simulink model "HDVSim_BEV_Truck"  (R2019b)
settings: Solver=ode3  StartTime=0.0  StopTime=inf  FixedStep=sample_time  MaxStep=0.1  RelTol=1e-3  EnableMultiTasking=on
model workspace (MAT data in the model file):
  Bat : object (value not decoded)
  Electric_Truck = 1
  FuelCell : P_nom (value not decoded)
  Fueltype = 7
  Hybrid_Truck = 1
  IZ12 = 3600
  M_el = 1000
  SOC_T_EM_completely_available = 0.5
  SOC_addition = 0.4
  SOC_el = 0.8
  SOC_target = 0.85
  Sailing_without_drag_torque = 0
  TCO : object (value not decoded)
  TCO_Trailer = 1
  T_distance_LPS_down = 250
  T_distance_LPS_up = 250
  VSim : object (value not decoded)
  Vehicle = 'empty'
  WPT : object (value not decoded)
  acquisitionCosts : acquisitionCosts (value not decoded)
  addition_for_critical_slope = 0.01
  ambient : object (value not decoded)
  auxiliary_consumers : object (value not decoded)
  critical_altitude_difference = 50
  cycle : object (value not decoded)
  dcycle = 22
  distance_1_PPC = 175
  distance_2_PPC = 200
  distance_PPC_altitude_difference = 10000
  driver : object (value not decoded)
  em : object (value not decoded)
  engine : object (value not decoded)
  final_drive : object (value not decoded)
  ifElectric = 1
  ifOptimized = 0
  look_ahead_PPC = 250
  max_distance = 100000
  name = 'HDVSim_BEV_Truck'
  preditiveCruiseControl = 0
  sample_time = 0.1
  tank : object (value not decoded)
  tires : object (value not decoded)
  transmission : object (value not decoded)
  v_PPC_delta = 2.77777777778
  v_max_electrical_drive_only = 13.8888888889
  vehicle : object (value not decoded)
  vehicleProperties : vehicleProperties (value not decoded)
  weights : weights (value not decoded)
  x = 1
values from neighbouring files (symbols this model uses):
  transmission = Transmission_gearing(15.86, 7, 0, 0, final_drive.ratio)    [Parameterizing.m]
symbols that are objects in the model workspace (value not decoded): ambient, auxiliary_consumers, Bat, cycle, driver, em, final_drive, tires, vehicle
undefined symbols (not defined in the file or in its folder): Ion, Lithium, prospective_cruise_control, Vorausschauender_Tempomat
libraries: simulink x21, powerlib x2, electricdrivelib x1
(part 2 of 3)

== system HDVSim_BEV_Truck/Active cruise control1/Estimate acceleration ==
  v_target [m/s] : Inport
  Slope_0 : Inport  Port=2
  Slope_50 : Inport  Port=3
  Slope_100 : Inport  Port=4
  Slope_150 : Inport  Port=5
  Slope_200 : Inport  Port=6
  "Slope_250 " : Inport  Port=7
  Slope_300 : Inport  Port=8
  Slope_350 : Inport  Port=9
  Slope_400 : Inport  Port=10
  Slope_450 : Inport  Port=11
  Add4 : Sum
  Constant4 : Constant  Value=vehicle.payload
  Constant9 : Constant  Value=vehicle.mass
  Demux : Demux  Outputs=10
  Divide1 : Product  Inputs=*/
  Driving resistance without acceleration : Subsystem
  Gain1 : Gain  Gain=-1
  Mux : Mux  Inputs=10
  Trigonometric Function2 : Trigonometry  Operator=atan
  Acceleration_0 : Outport  VectorParamsAs1DForOutWhenUnconnected=off
  Acceleration_50 : Outport  Port=2  VectorParamsAs1DForOutWhenUnconnected=off
  Acceleration_100 : Outport  Port=3  VectorParamsAs1DForOutWhenUnconnected=off
  Acceleration_150 : Outport  Port=4  VectorParamsAs1DForOutWhenUnconnected=off
  Acceleration_200 : Outport  Port=5  VectorParamsAs1DForOutWhenUnconnected=off
  Acceleration_250 : Outport  Port=6  VectorParamsAs1DForOutWhenUnconnected=off
  Acceleration_300 : Outport  Port=7  VectorParamsAs1DForOutWhenUnconnected=off
  Acceleration_350 : Outport  Port=8  VectorParamsAs1DForOutWhenUnconnected=off
  Acceleration_400 : Outport  Port=9  VectorParamsAs1DForOutWhenUnconnected=off
  Acceleration_450 : Outport  Port=10  VectorParamsAs1DForOutWhenUnconnected=off
  wires:
  v_target [m/s]/1 -> Driving resistance without acceleration/1(v [m/s])
  Trigonometric Function2/1 -> Driving resistance without acceleration/2(alpha [rad])
  Constant9/1 -> Add4/1
  Constant4/1 -> Add4/2
  Driving resistance without acceleration/1(F_x (resist) [N]) -> Gain1/1
  Add4/1 -> Divide1/2
  Gain1/1 -> Divide1/1
  Mux/1 -> Trigonometric Function2/1
  Divide1/1 -> Demux/1
  Demux/1 -> Acceleration_0/1
  Slope_0/1 -> Mux/1
  Slope_50/1 -> Mux/2
  Slope_100/1 -> Mux/3
  Slope_150/1 -> Mux/4
  Slope_200/1 -> Mux/5
  "Slope_250 "/1 -> Mux/6
  Slope_300/1 -> Mux/7
  Slope_350/1 -> Mux/8
  Slope_400/1 -> Mux/9
  Slope_450/1 -> Mux/10
  Demux/2 -> Acceleration_50/1
  Demux/3 -> Acceleration_100/1
  Demux/4 -> Acceleration_150/1
  Demux/5 -> Acceleration_200/1
  Demux/6 -> Acceleration_250/1
  Demux/7 -> Acceleration_300/1
  Demux/8 -> Acceleration_350/1
  Demux/9 -> Acceleration_400/1
  Demux/10 -> Acceleration_450/1

== system HDVSim_BEV_Truck/Active cruise control1/Estimate critical slope ==
  note: Total resistive forces on the vehicle
  note: Friction resistance
  note: Drag on the vehicle
  note: Forward force applied on the vehicle
  v_target [m/s] : Inport
  A : Constant  Value=vehicle.frontal_area
  Add : Sum
  Add1 : Sum
  Constant1 : Constant  Value=vehicle.payload
  Constant4 : Constant  Value=addition_for_critical_slope
  Constant5 : Constant  Value=tires.roll_drag_coeff.total
  Constant8 : Constant  Value=vehicle.mass
  Differential gear ratio : Constant  Value=final_drive.ratio
  Divide : Product  Inputs=***/
  Divide1 : Product  Inputs=*/
  Gain : Gain  Gain=0.95
  Product : Product
  Product2 : Product  Inputs=4  RndMeth=Zero
  Saturation : Saturate  UpperLimit=1  LowerLimit=-1
  Subtract : Sum  Inputs=+-
  Sum3 : Sum  Inputs=++|
  Tire radius : Constant  Value=tires.radius
  Trigonometric Function : Trigonometry  Operator=asin
  Trigonometric Function1 : Trigonometry  Operator=tan
  c_d : Constant  Value=vehicle.air_drag_coeff(end)
  g : Gain  Gain=ambient.gravity
  gain2 : Gain  Gain=0.5
  rho : Constant  Value=ambient.air_density
  v² : Math  Operator=square  SaturateOnIntegerOverflow=on
  critical_slope : Outport  VectorParamsAs1DForOutWhenUnconnected=off
  wires:
  Subtract/1 -> Divide1/1  "F_net"
  v²/1 -> Product2/1
  rho/1 -> Product2/2
  A/1 -> Product2/3
  c_d/1 -> Product2/4
  Product2/1 -> gain2/1
  Constant8/1 -> Add1/1
  Constant1/1 -> Add1/2
  Add1/1 -> g/1
  Constant5/1 -> Product/2
  Trigonometric Function/1 -> Trigonometric Function1/1
  Divide1/1 -> Saturation/1
  Sum3/1 -> critical_slope/1
  Constant4/1 -> Sum3/1
  Trigonometric Function1/1 -> Sum3/2
  v_target [m/s]/1 -> v²/1
  gain2/1 -> Add/1
  Product/1 -> Add/2
  Add/1 -> Subtract/2  "F_resistive"
  g/1 -> Product/1, Divide1/2
  Saturation/1 -> Trigonometric Function/1
  Tire radius/1 -> Divide/4
  Differential gear ratio/1 -> Divide/2
  Gain/1 -> Divide/3
  [i_gearbox] -> Divide/1
  Divide/1 -> Subtract/1
  [M_EM_max] -> Gain/1

== system HDVSim_BEV_Truck/Active cruise control2/Braking from upper speed limit ==
  v_target [m/s] : Inport
  Add3 : Sum  Inputs=+-
  Constant1 : Constant  Value=90/3.6
  Constant10 : Constant  Value=preditiveCruiseControl
  Constant6 : Constant  Value=v_PPC_delta
  Constant7 : Constant  Value=0
  Constant8 : Constant  Value=0
  Saturation Dynamic : simulink/Discontinuities/Saturation Dynamic  OutMin=[]  OutMax=[]  OutDataTypeStr=Inherit: Same as second input  OutDataType=fixdt(1, 16)  OutScaling=2^-10  DoSatur=off
  Switch3 : Switch  Criteria=u2 > Threshold
  Out1 : Outport  VectorParamsAs1DForOutWhenUnconnected=off
  wires:
  Switch3/1 -> Out1/1
  Constant6/1 -> Saturation Dynamic/2
  Constant1/1 -> Add3/1
  Constant7/1 -> Switch3/3
  Add3/1 -> Saturation Dynamic/1
  Constant8/1 -> Saturation Dynamic/3
  Constant10/1 -> Switch3/2
  v_target [m/s]/1 -> Add3/2
  Saturation Dynamic/1 -> Switch3/1

== system HDVSim_BEV_Truck/Active cruise control2/Estimate acceleration ==
  v_target [m/s] : Inport
  Slope_0 : Inport  Port=2
  Slope_50 : Inport  Port=3
  Slope_100 : Inport  Port=4
  Slope_150 : Inport  Port=5
  Slope_200 : Inport  Port=6
  "Slope_250 " : Inport  Port=7
  Slope_300 : Inport  Port=8
  Slope_350 : Inport  Port=9
  Slope_400 : Inport  Port=10
  Slope_450 : Inport  Port=11
  Add4 : Sum
  Constant4 : Constant  Value=vehicle.payload
  Constant9 : Constant  Value=vehicle.mass
  Demux : Demux  Outputs=10
  Divide1 : Product  Inputs=*/
  Driving resistance without acceleration : Subsystem
  Gain1 : Gain  Gain=-1
  Mux : Mux  Inputs=10
  Trigonometric Function2 : Trigonometry  Operator=atan
  Acceleration_0 : Outport  VectorParamsAs1DForOutWhenUnconnected=off
  Acceleration_50 : Outport  Port=2  VectorParamsAs1DForOutWhenUnconnected=off
  Acceleration_100 : Outport  Port=3  VectorParamsAs1DForOutWhenUnconnected=off
  Acceleration_150 : Outport  Port=4  VectorParamsAs1DForOutWhenUnconnected=off
  Acceleration_200 : Outport  Port=5  VectorParamsAs1DForOutWhenUnconnected=off
  Acceleration_250 : Outport  Port=6  VectorParamsAs1DForOutWhenUnconnected=off
  Acceleration_300 : Outport  Port=7  VectorParamsAs1DForOutWhenUnconnected=off
  Acceleration_350 : Outport  Port=8  VectorParamsAs1DForOutWhenUnconnected=off
  Acceleration_400 : Outport  Port=9  VectorParamsAs1DForOutWhenUnconnected=off
  Acceleration_450 : Outport  Port=10  VectorParamsAs1DForOutWhenUnconnected=off
  wires:
  v_target [m/s]/1 -> Driving resistance without acceleration/1(v [m/s])
  Trigonometric Function2/1 -> Driving resistance without acceleration/2(alpha [rad])
  Constant9/1 -> Add4/1
  Constant4/1 -> Add4/2
  Driving resistance without acceleration/1(F_x (resist) [N]) -> Gain1/1
  Add4/1 -> Divide1/2
  Gain1/1 -> Divide1/1
  Mux/1 -> Trigonometric Function2/1
  Divide1/1 -> Demux/1
  Demux/1 -> Acceleration_0/1
  Slope_0/1 -> Mux/1
  Slope_50/1 -> Mux/2
  Slope_100/1 -> Mux/3
  Slope_150/1 -> Mux/4
  Slope_200/1 -> Mux/5
  "Slope_250 "/1 -> Mux/6
  Slope_300/1 -> Mux/7
  Slope_350/1 -> Mux/8
  Slope_400/1 -> Mux/9
  Slope_450/1 -> Mux/10
  Demux/2 -> Acceleration_50/1
  Demux/3 -> Acceleration_100/1
  Demux/4 -> Acceleration_150/1
  Demux/5 -> Acceleration_200/1
  Demux/6 -> Acceleration_250/1
  Demux/7 -> Acceleration_300/1
  Demux/8 -> Acceleration_350/1
  Demux/9 -> Acceleration_400/1
  Demux/10 -> Acceleration_450/1

== system HDVSim_BEV_Truck/Active cruise control2/Estimate critical slope ==
  note: Total resistive forces on the vehicle
  note: Friction resistance
  note: Drag on the vehicle
  note: Forward force applied on the vehicle
  v_target [m/s] : Inport
  A : Constant  Value=vehicle.frontal_area
  Add : Sum
  Add1 : Sum
  Add3 : Sum
  Constant1 : Constant  Value=vehicle.payload
  Constant4 : Constant  Value=addition_for_critical_slope
  Constant5 : Constant  Value=tires.roll_drag_coeff.total
  Constant8 : Constant  Value=vehicle.mass
  Differential efficiency : Constant  Value=final_drive.trq_eff
  Differential gear ratio : Constant  Value=final_drive.ratio
  Divide : Product  Inputs=***/**
  Divide1 : Product  Inputs=*/
  Product : Product
  Product2 : Product  Inputs=4  RndMeth=Zero
  Subtract : Sum  Inputs=+-
  Sum3 : Sum  Inputs=++|
  Tire radius : Constant  Value=tires.radius
  Trigonometric Function : Trigonometry  Operator=asin
  Trigonometric Function1 : Trigonometry  Operator=tan
  c_d : Constant  Value=vehicle.air_drag_coeff(end)
  g : Gain  Gain=ambient.gravity
  gain2 : Gain  Gain=0.5
  rho : Constant  Value=ambient.air_density
  v² : Math  Operator=square  SaturateOnIntegerOverflow=on
  critical_slope : Outport  VectorParamsAs1DForOutWhenUnconnected=off
  wires:
  Add3/1 -> Divide/3
  [i_gearbox] -> Divide/1
  Differential gear ratio/1 -> Divide/2
  Tire radius/1 -> Divide/4
  Divide/1 -> Subtract/1
  Subtract/1 -> Divide1/1  "F_net"
  v²/1 -> Product2/1
  rho/1 -> Product2/2
  A/1 -> Product2/3
  c_d/1 -> Product2/4
  Product2/1 -> gain2/1
  Constant8/1 -> Add1/1
  Constant1/1 -> Add1/2
  Add1/1 -> g/1
  Constant5/1 -> Product/2
  Trigonometric Function/1 -> Trigonometric Function1/1
  Divide1/1 -> Trigonometric Function/1
  Sum3/1 -> critical_slope/1
  Constant4/1 -> Sum3/1
  Trigonometric Function1/1 -> Sum3/2
  v_target [m/s]/1 -> v²/1
  [Eta_Transmission] -> Divide/5
  Differential efficiency/1 -> Divide/6
  [M_EM_max] -> Add3/1
  [M_EM_max] -> Add3/2
  gain2/1 -> Add/1
  Product/1 -> Add/2
  Add/1 -> Subtract/2  "F_resistive"
  g/1 -> Product/1, Divide1/2

== system HDVSim_BEV_Truck/Active cruise control_old/Braking from upper speed limit ==
  v_soll [m/s] : Inport
  Add3 : Sum  Inputs=+-
  Constant1 : Constant  Value=90/3.6
  Constant10 : Constant  Value=Vorausschauender_Tempomat
  Constant6 : Constant  Value=6/3.6
  Constant7 : Constant  Value=0
  Constant8 : Constant  Value=0
  Saturation Dynamic : simulink/Discontinuities/Saturation Dynamic  OutMin=[]  OutMax=[]  OutDataTypeStr=Inherit: Same as second input  OutDataType=fixdt(1, 16)  OutScaling=2^-10  DoSatur=off
  Switch3 : Switch  Criteria=u2 > Threshold
  Out1 : Outport  VectorParamsAs1DForOutWhenUnconnected=off
  wires:
  Switch3/1 -> Out1/1
  Constant6/1 -> Saturation Dynamic/2
  Constant1/1 -> Add3/1
  Constant7/1 -> Switch3/3
  Add3/1 -> Saturation Dynamic/1
  Constant8/1 -> Saturation Dynamic/3
  Constant10/1 -> Switch3/2
  v_soll [m/s]/1 -> Add3/2
  Saturation Dynamic/1 -> Switch3/1

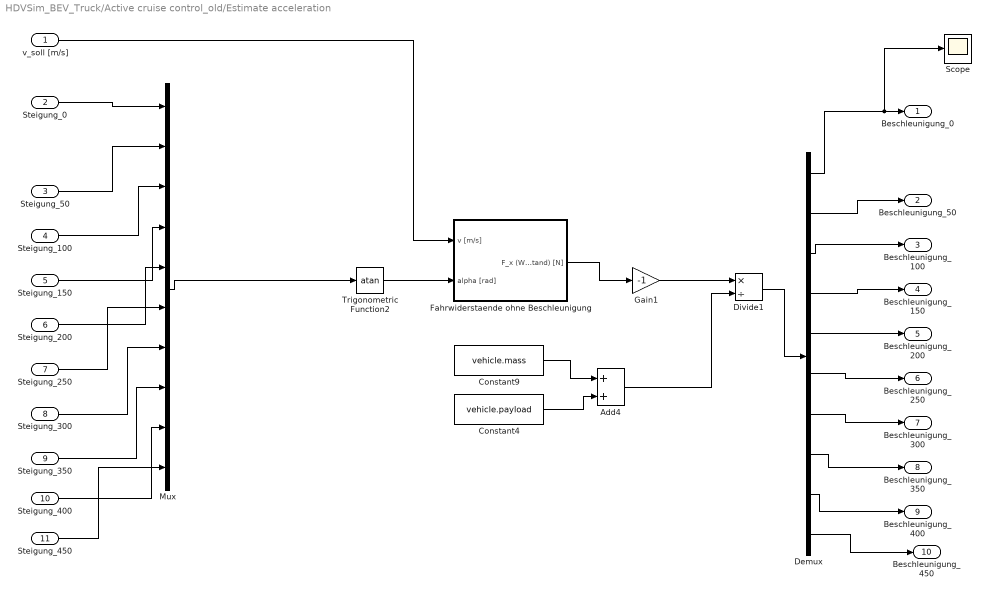
== system HDVSim_BEV_Truck/Active cruise control_old/Estimate acceleration ==
  v_soll [m/s] : Inport
  Steigung_0 : Inport  Port=2
  Steigung_50 : Inport  Port=3
  Steigung_100 : Inport  Port=4
  Steigung_150 : Inport  Port=5
  Steigung_200 : Inport  Port=6
  "Steigung_250 " : Inport  Port=7
  Steigung_300 : Inport  Port=8
  Steigung_350 : Inport  Port=9
  Steigung_400 : Inport  Port=10
  Steigung_450 : Inport  Port=11
  Add4 : Sum
  Constant4 : Constant  Value=vehicle.payload
  Constant9 : Constant  Value=vehicle.mass
  Demux : Demux  Outputs=10
  Divide1 : Product  Inputs=*/
  Fahrwiderstaende ohne Beschleunigung : Subsystem
  Gain1 : Gain  Gain=-1
  Mux : Mux  Inputs=10
  Scope : Scope
  Trigonometric Function2 : Trigonometry  Operator=atan
  Beschleunigung_0 : Outport  VectorParamsAs1DForOutWhenUnconnected=off
  Beschleunigung_50 : Outport  Port=2  VectorParamsAs1DForOutWhenUnconnected=off
  Beschleunigung_100 : Outport  Port=3  VectorParamsAs1DForOutWhenUnconnected=off
  Beschleunigung_150 : Outport  Port=4  VectorParamsAs1DForOutWhenUnconnected=off
  Beschleunigung_200 : Outport  Port=5  VectorParamsAs1DForOutWhenUnconnected=off
  Beschleunigung_250 : Outport  Port=6  VectorParamsAs1DForOutWhenUnconnected=off
  Beschleunigung_300 : Outport  Port=7  VectorParamsAs1DForOutWhenUnconnected=off
  Beschleunigung_350 : Outport  Port=8  VectorParamsAs1DForOutWhenUnconnected=off
  Beschleunigung_400 : Outport  Port=9  VectorParamsAs1DForOutWhenUnconnected=off
  Beschleunigung_450 : Outport  Port=10  VectorParamsAs1DForOutWhenUnconnected=off
  wires:
  v_soll [m/s]/1 -> Fahrwiderstaende ohne Beschleunigung/1(v [m/s])
  Trigonometric Function2/1 -> Fahrwiderstaende ohne Beschleunigung/2(alpha [rad])
  Constant9/1 -> Add4/1
  Constant4/1 -> Add4/2
  Fahrwiderstaende ohne Beschleunigung/1(F_x (Widerstand) [N]) -> Gain1/1
  Add4/1 -> Divide1/2
  Gain1/1 -> Divide1/1
  Mux/1 -> Trigonometric Function2/1
  Divide1/1 -> Demux/1
  Demux/1 -> Scope/1, Beschleunigung_0/1
  Steigung_0/1 -> Mux/1
  Steigung_50/1 -> Mux/2
  Steigung_100/1 -> Mux/3
  Steigung_150/1 -> Mux/4
  Steigung_200/1 -> Mux/5
  "Steigung_250 "/1 -> Mux/6
  Steigung_300/1 -> Mux/7
  Steigung_350/1 -> Mux/8
  Steigung_400/1 -> Mux/9
  Steigung_450/1 -> Mux/10
  Demux/2 -> Beschleunigung_50/1
  Demux/3 -> Beschleunigung_100/1
  Demux/4 -> Beschleunigung_150/1
  Demux/5 -> Beschleunigung_200/1
  Demux/6 -> Beschleunigung_250/1
  Demux/7 -> Beschleunigung_300/1
  Demux/8 -> Beschleunigung_350/1
  Demux/9 -> Beschleunigung_400/1
  Demux/10 -> Beschleunigung_450/1

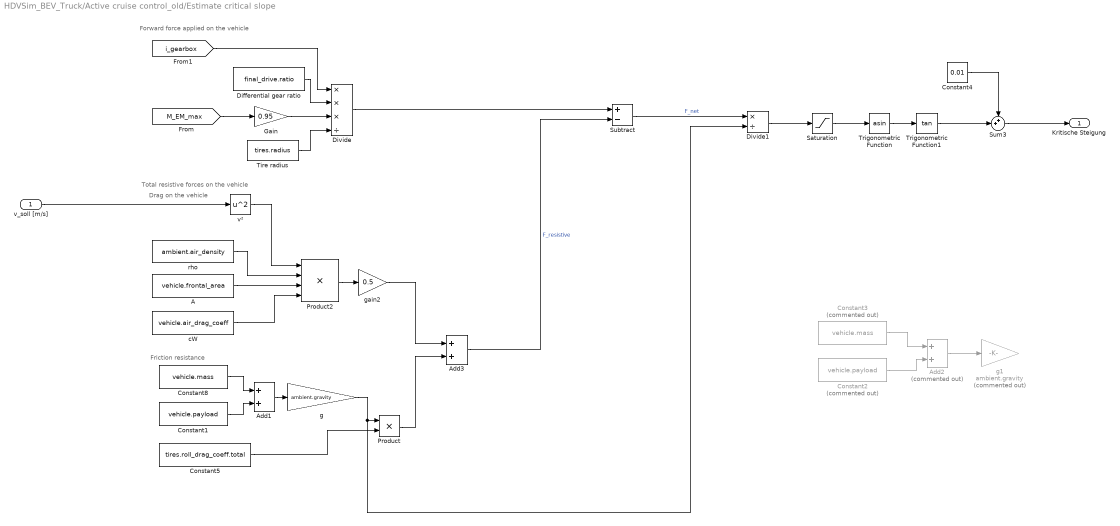
== system HDVSim_BEV_Truck/Active cruise control_old/Estimate critical slope ==
  note: Forward force applied on the vehicle
  note: Total resistive forces on the vehicle
  note: Drag on the vehicle
  note: Friction resistance
  v_soll [m/s] : Inport
  A : Constant  Value=vehicle.frontal_area
  Add1 : Sum
  Add2 : Sum  Commented=on
  Add3 : Sum
  Constant1 : Constant  Value=vehicle.payload
  Constant2 : Constant  Commented=on  Value=vehicle.payload
  Constant3 : Constant  Commented=on  Value=vehicle.mass
  Constant4 : Constant  Value=0.01
  Constant5 : Constant  Value=tires.roll_drag_coeff.total
  Constant8 : Constant  Value=vehicle.mass
  Differential gear ratio : Constant  Value=final_drive.ratio
  Divide : Product  Inputs=***/
  Divide1 : Product  Inputs=*/
  Gain : Gain  Gain=0.95
  Product : Product
  Product2 : Product  Inputs=4  RndMeth=Zero
  Saturation : Saturate  UpperLimit=1  LowerLimit=-1
  Subtract : Sum  Inputs=+-
  Sum3 : Sum  Inputs=++|
  Tire radius : Constant  Value=tires.radius
  Trigonometric Function : Trigonometry  Operator=asin
  Trigonometric Function1 : Trigonometry  Operator=tan
  cW : Constant  Value=vehicle.air_drag_coeff
  g : Gain  Gain=ambient.gravity
  g1 : Gain  Commented=on  Gain=ambient.gravity
  gain2 : Gain  Gain=0.5
  rho : Constant  Value=ambient.air_density
  v² : Math  Operator=square  SaturateOnIntegerOverflow=on
  Kritische Steigung : Outport  VectorParamsAs1DForOutWhenUnconnected=off
  wires:
  Gain/1 -> Divide/3
  [i_gearbox] -> Divide/1
  Differential gear ratio/1 -> Divide/2
  Tire radius/1 -> Divide/4
  Divide/1 -> Subtract/1
  v²/1 -> Product2/1
  rho/1 -> Product2/2
  A/1 -> Product2/3
  cW/1 -> Product2/4
  Product2/1 -> gain2/1
  Constant8/1 -> Add1/1
  Constant1/1 -> Add1/2
  Add1/1 -> g/1
  Constant5/1 -> Product/2
  Constant3/1 -> Add2/1
  Constant2/1 -> Add2/2
  Add2/1 -> g1/1
  Trigonometric Function/1 -> Trigonometric Function1/1
  Divide1/1 -> Saturation/1
  Sum3/1 -> Kritische Steigung/1
  [M_EM_max] -> Gain/1
  Constant4/1 -> Sum3/1
  Trigonometric Function1/1 -> Sum3/2
  v_soll [m/s]/1 -> v²/1
  Saturation/1 -> Trigonometric Function/1
  gain2/1 -> Add3/1
  Product/1 -> Add3/2
  Subtract/1 -> Divide1/1  "F_net"
  Add3/1 -> Subtract/2  "F_resistive"
  g/1 -> Product/1, Divide1/2

== system HDVSim_BEV_Truck/Driver controls/PI controller brake1 ==
  delta_v : Inport
  Add : Sum
  "I - controller " : Gain  Gain=driver.controller_integral_gain
  "Integrator, reset for sign change of delta v" : Integrator  ExternalReset=either  ZeroCross=off
  "P - controller " : Gain  Gain=driver.controller_proportional_gain
  F_target [N] : Outport  VectorParamsAs1DForOutWhenUnconnected=off
  wires:
  "Integrator, reset for sign change of delta v"/1 -> Add/2  "I_part"
  "I - controller "/1 -> "Integrator, reset for sign change of delta v"/1
  Add/1 -> F_target [N]/1  "F_target"
  "P - controller "/1 -> Add/1  "P_part"
  delta_v/1 -> "I - controller "/1, "Integrator, reset for sign change of delta v"/2, "P - controller "/1

== system HDVSim_BEV_Truck/Driver controls/PI controller throttle1 ==
  delta_v : Inport
  Add : Sum
  "I - controller " : Gain  Gain=driver.controller_integral_gain
  "Integrator, reset for sign change of delta v" : Integrator  ExternalReset=either  ZeroCross=off
  "P - controller " : Gain  Gain=driver.controller_proportional_gain
  F_target [N] : Outport  VectorParamsAs1DForOutWhenUnconnected=off
  wires:
  "Integrator, reset for sign change of delta v"/1 -> Add/2  "I_part"
  "I - controller "/1 -> "Integrator, reset for sign change of delta v"/1
  Add/1 -> F_target [N]/1  "F_target"
  "P - controller "/1 -> Add/1  "P_partl"
  delta_v/1 -> "Integrator, reset for sign change of delta v"/2, "I - controller "/1, "P - controller "/1

== system HDVSim_BEV_Truck/Driver controls/ZKU ==
  In1 : Inport
  Switch1 : Switch  Threshold=1
  zero1 : Constant  Value=0
  Out1 : Outport  VectorParamsAs1DForOutWhenUnconnected=off
  wires:
  zero1/1 -> Switch1/1
  [ZKU] -> Switch1/2
  Switch1/1 -> Out1/1
  In1/1 -> Switch1/3

== system HDVSim_BEV_Truck/Driver controls/ZKU1 ==
  In1 : Inport
  Switch1 : Switch  Threshold=1
  zero1 : Constant  Value=0
  Out1 : Outport  VectorParamsAs1DForOutWhenUnconnected=off
  wires:
  In1/1 -> Switch1/3
  Switch1/1 -> Out1/1
  [ZKU] -> Switch1/2
  zero1/1 -> Switch1/1

== system HDVSim_BEV_Truck/Driving cycle/Holding time at the beginning ==
  In1 : Inport
  Clock2 : Clock
  Constant3 : Constant  Value=cycle.stop_start
  Constant4 : Constant  Value=0
  Subtract1 : Sum  Inputs=+-
  Switch1 : Switch
  Out1 : Outport  VectorParamsAs1DForOutWhenUnconnected=off
  wires:
  In1/1 -> Switch1/1
  Constant3/1 -> Subtract1/2
  Clock2/1 -> Subtract1/1
  Constant4/1 -> Switch1/3
  Subtract1/1 -> Switch1/2
  Switch1/1 -> Out1/1

== system HDVSim_BEV_Truck/Driving cycle/Holding time at the end ==
  In1 : Inport
  Clock1 : Clock
  Constant : Constant
  Constant1 : Constant  Value=cycle.stop_end
  Constant2 : Constant
  Hit Crossing : HitCross  HitCrossingDirection=rising
  Integrator : Integrator  ExternalReset=rising
  Subtract : Sum  Inputs=+-
  Sum1 : Sum  Inputs=|++
  Switch : Switch  Criteria=u2 > Threshold  Threshold=cycle.stop_end
  Out1 : Outport  VectorParamsAs1DForOutWhenUnconnected=off
  wires:
  In1/1 -> Integrator/2
  Constant/1 -> Integrator/1
  Subtract/1 -> Hit Crossing/1
  Integrator/1 -> Switch/1
  Hit Crossing/1 -> Out1/1
  Clock1/1 -> Switch/2
  Constant1/1 -> Sum1/2, Subtract/2
  Sum1/1 -> Switch/3
  Switch/1 -> Subtract/1
  Constant2/1 -> Sum1/1

== system HDVSim_BEV_Truck/Driving cycle/Significant speed deviation ==
  In1 : Inport
  Clock : Clock
  Compare To Constant : simulink/Logic and Bit Operations/Compare To Constant  relop=>=  const=30  OutDataTypeStr=boolean
  Compare To Constant1 : simulink/Logic and Bit Operations/Compare To Constant  relop=>=  const=1000  OutDataTypeStr=boolean
  Compare To Constant2 : simulink/Logic and Bit Operations/Compare To Constant  relop=<=  const=0.1  OutDataTypeStr=boolean
  Compare To Constant3 : simulink/Logic and Bit Operations/Compare To Constant  relop=>=  const=1000  OutDataTypeStr=boolean
  Constant : Constant
  Constant1 : Constant  Value=0
  Constant2 : Constant
  Constant3 : Constant  Value=0
  Display : Display
  Display1 : Display
  Display2 : Display
  Gain : Gain  Gain=3.6
  Gain1 : Gain  Gain=3.6
  Integrator1 : Integrator  ExternalReset=either
  Integrator2 : Integrator  ExternalReset=either
  Logical Operator : Logic  Operator=OR  AllPortsSameDT=off  OutDataTypeStr=boolean
  Scope : Scope
  Sum : Sum  Inputs=|+-
  Switch : Switch  Criteria=u2 > Threshold
  Switch1 : Switch  Criteria=u2 > Threshold
  stop_time : Lookup_n-D  NumberOfTableDimensions=1  BreakpointsForDimension1=cycle.distance  Table=cycle.stop_time  InterpMethod=Flat  RndMeth=Simplest  InputSameDT=on
  Out1 : Outport  VectorParamsAs1DForOutWhenUnconnected=off
  wires:
  In1/1 -> stop_time/1
  stop_time/1 -> Scope/1, Sum/2
  [delta_v] -> Gain/1
  [v_current1] -> Gain1/1
  Gain/1 -> Compare To Constant/1
  Integrator2/1 -> Display/1, Compare To Constant1/1
  Compare To Constant1/1 -> Logical Operator/2
  Gain1/1 -> Compare To Constant2/1
  Integrator1/1 -> Sum/1
  Sum/1 -> Display1/1, Compare To Constant3/1
  Compare To Constant3/1 -> Logical Operator/1
  Logical Operator/1 -> Out1/1
  Switch1/1 -> Integrator2/1, Integrator2/2
  Switch/1 -> Integrator1/2, Integrator1/1
  Constant/1 -> Switch/1
  Compare To Constant2/1 -> Switch/2
  Constant1/1 -> Switch/3
  Constant2/1 -> Switch1/1
  Compare To Constant/1 -> Switch1/2
  Constant3/1 -> Switch1/3
  Clock/1 -> Display2/1

== system HDVSim_BEV_Truck/ECU/Approach to stop ==
  stop_time [s] : Inport
  Add : Sum  Inputs=+-
  Clock : Clock
  Compare To Constant1 : simulink/Logic and Bit Operations/Compare To Constant  relop=<=  const=8  OutDataTypeStr=boolean
  Compare To Zero : simulink/Logic and Bit Operations/Compare To Zero  relop=<=  OutDataTypeStr=boolean
  Constant : Constant
  Constant1 : Constant  Value=4
  Constant2 : Constant
  Display : Display
  Hit Crossing : HitCross  HitCrossingDirection=rising
  Integrator : Integrator  ExternalReset=rising  InitialCondition=0.001
  Integrator1 : Integrator  ExternalReset=rising
  Scope : Scope  NumInputPorts=4
  Subtract : Sum  Inputs=+-
  Switch : Switch  Criteria=u2 > Threshold  Threshold=14
  Driver_M : Outport  VectorParamsAs1DForOutWhenUnconnected=off
  Driver_B : Outport  Port=2  VectorParamsAs1DForOutWhenUnconnected=off
  wires:
  Constant/1 -> Integrator/1
  stop_time [s]/1 -> Integrator/2, Add/2, Scope/3, Subtract/2
  Integrator/1 -> Scope/4, Subtract/1
  Subtract/1 -> Compare To Zero/1, Hit Crossing/1
  Constant2/1 -> Integrator1/1
  Hit Crossing/1 -> Integrator1/2
  Constant1/1 -> Switch/3
  Integrator1/1 -> Switch/1
  Switch/1 -> Compare To Constant1/1
  Compare To Constant1/1 -> Scope/1, Driver_M/1
  Compare To Zero/1 -> Scope/2, Driver_B/1
  Clock/1 -> Add/1
  Add/1 -> Switch/2, Display/1

== system HDVSim_BEV_Truck/ECU/Calculations for braking ==
  note: Breaking from disk brakes
  note: Breaking from motor's regenerative breaking
  M_EM_max [Nm] : Inport
  Driver_B : Inport  Port=2
  Gear : Inport  Port=3
  Differential efficiency : Constant  Value=final_drive.trq_eff
  Differential gear ratio : Constant  Value=final_drive.ratio
  Divide : Product  Inputs=*/
  Divide1 : Product  Inputs=**/*/
  Efficiencies : Lookup  InputValues=[1:length(transmission.ratios)]  Table=transmission.trq_eff  LookUpMeth=Use Input Nearest
  Gearing : Lookup  InputValues=[1:length(transmission.ratios)]  Table=transmission.ratios  LookUpMeth=Use Input Nearest
  Maximum breaking force [N] : Constant  Value=vehicle.F_brake_max
  Product : Product
  Tire radius : Constant  Value=tires.radius
  F_brake_required [N] : Outport  VectorParamsAs1DForOutWhenUnconnected=off
  F_brake_elec_max [N] : Outport  Port=2  VectorParamsAs1DForOutWhenUnconnected=off
  wires:
  M_EM_max [Nm]/1 -> Divide1/1
  Divide/1 -> F_brake_elec_max [N]/1
  Divide1/1 -> Divide/1
  Tire radius/1 -> Divide/2
  Driver_B/1 -> Product/1
  Maximum breaking force [N]/1 -> Product/2
  Product/1 -> F_brake_required [N]/1
  Gear/1 -> Efficiencies/1, Gearing/1
  Gearing/1 -> Divide1/2
  Efficiencies/1 -> Divide1/3
  Differential gear ratio/1 -> Divide1/4
  Differential efficiency/1 -> Divide1/5

== system HDVSim_BEV_Truck/ECU/Calculations for throttle ==
  Driver_M : Inport
  SOC : Inport  Port=2
  n_EM [rpm] : Inport  Port=3
  Electrical machine speed-torque characteristics : Lookup_n-D  NumberOfTableDimensions=1  BreakpointsForDimension1=em.speed  Table=em.trq  ExtrapMethod=Clip  UseLastTableValue=on  RndMeth=Simplest  InputSameDT=on
  Memory1 : Memory
  Product : Product
  Product1 : Product
  M_EM_max [Nm] : Outport  VectorParamsAs1DForOutWhenUnconnected=off
  M_Required [Nm] : Outport  Port=2  VectorParamsAs1DForOutWhenUnconnected=off
  wires:
  Product1/1 -> Product/2
  Driver_M/1 -> Product/1
  Product/1 -> M_Required [Nm]/1
  Electrical machine speed-torque characteristics/1 -> Product1/1, M_EM_max [Nm]/1
  SOC/1 -> Product1/2
  n_EM [rpm]/1 -> Memory1/1
  Memory1/1 -> Electrical machine speed-torque characteristics/1

== system HDVSim_BEV_Truck/Electric motor/Machine current demand ==
  note: Electric power calculation
  "n_EM " : Inport
  M_EM_target [Nm] : Inport  Port=2
  Eff_EM : Inport  Port=3
  U_Bat [V] : Inport  Port=4
  Divide : Product  Inputs=*/*
  Divide1 : Product  Inputs=*/
  Gain : Gain  Gain=2*pi/60
  Saturation1 : Saturate  UpperLimit=inf  LowerLimit=1
  I_target [A] : Outport  VectorParamsAs1DForOutWhenUnconnected=off
  wires:
  Divide/1 -> Divide1/1
  Divide1/1 -> I_target [A]/1
  Gain/1 -> Divide/3
  M_EM_target [Nm]/1 -> Divide/1
  "n_EM "/1 -> Saturation1/1
  U_Bat [V]/1 -> Divide1/2
  Eff_EM/1 -> Divide/2
  Saturation1/1 -> Gain/1

== system HDVSim_BEV_Truck/Electric motor/Machine torque demand ==
  n_EM [rpm] : Inport
  I_current [A] : Inport  Port=2
  Eff_EM : Inport  Port=3
  U_Bat [V] : Inport  Port=4
  Divide : Product  Inputs=*/*
  Gain : Gain  Gain=2*pi/60
  Product : Product
  Saturation1 : Saturate  UpperLimit=em.n_max  LowerLimit=1
  M_EM [Nm] : Outport  VectorParamsAs1DForOutWhenUnconnected=off
  wires:
  U_Bat [V]/1 -> Product/1
  n_EM [rpm]/1 -> Saturation1/1
  Product/1 -> Divide/1
  Gain/1 -> Divide/2
  Divide/1 -> M_EM [Nm]/1
  I_current [A]/1 -> Product/2
  Eff_EM/1 -> Divide/3
  Saturation1/1 -> Gain/1

== system HDVSim_BEV_Truck/Power electronics & battery/Conversion of SOC ==
  SOC_absolut : Inport
  Constant : Constant  Value=0.5-Bat.Useable_range/2
  Constant1 : Constant  Value=0.5+Bat.Useable_range/2
  Divide : Product  Inputs=*/
  Saturation : Saturate  UpperLimit=1  LowerLimit=0
  Sum : Sum  Inputs=+-
  Sum1 : Sum  Inputs=-+
  SOC_relative : Outport  VectorParamsAs1DForOutWhenUnconnected=off
  wires:
  SOC_absolut/1 -> Sum/1
  Constant/1 -> Sum1/1, Sum/2
  Sum/1 -> Divide/1
  Constant1/1 -> Sum1/2
  Sum1/1 -> Divide/2
  Divide/1 -> Saturation/1
  Saturation/1 -> SOC_relative/1

== system HDVSim_BEV_Truck/Power electronics & battery/Power electronics ==
  I_PE_current [A] : Inport
  1/Eta_LE : Gain  Gain=1/Bat.Efficiency_power_electronics
  Eta_LE : Gain  Gain=Bat.Efficiency_power_electronics
  Switch : Switch  Criteria=u2 > Threshold
  I_BAT_current [A] : Outport  VectorParamsAs1DForOutWhenUnconnected=off
  wires:
  Eta_LE/1 -> Switch/1
  1/Eta_LE/1 -> Switch/3
  I_PE_current [A]/1 -> 1/Eta_LE/1, Eta_LE/1, Switch/2
  Switch/1 -> I_BAT_current [A]/1

== system HDVSim_BEV_Truck/Power electronics & battery/To prevent division by zero ==
  In1 : Inport
  In2 : Inport  Port=2
  In3 : Inport  Port=3
  Enable : EnablePort
  Abs : Abs
  Divide1 : Product  Inputs=*/
  Product1 : Product
  Out1 : Outport  VectorParamsAs1DForOutWhenUnconnected=off
  wires:
  In2/1 -> Product1/1
  In1/1 -> Product1/2
  In3/1 -> Divide1/1
  Product1/1 -> Divide1/2
  Divide1/1 -> Abs/1
  Abs/1 -> Out1/1  "Losses (%)"

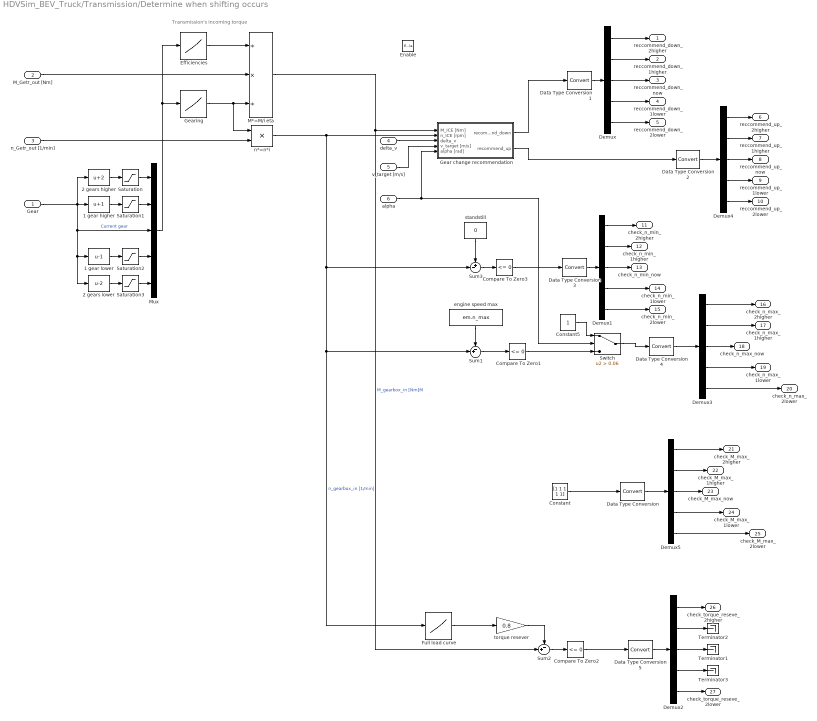
== system HDVSim_BEV_Truck/Transmission/Determine when shifting occurs ==
  note: Transmission's incoming torque
  Gear : Inport
  M_Getr_out [Nm] : Inport  Port=2
  n_Getr_out [1/min] : Inport  Port=3
  delta_v : Inport  Port=4
  v_target [m/s] : Inport  Port=5
  alpha : Inport  Port=6
  Enable : EnablePort
  1 gear higher : Bias  Bias=1
  1 gear lower : Bias  Bias=-1
  2 gears higher : Bias  Bias=2
  2 gears lower : Bias  Bias=-2
  Compare To Zero1 : simulink/Logic and Bit Operations/Compare To Zero  relop=<=  OutDataTypeStr=boolean
  Compare To Zero2 : simulink/Logic and Bit Operations/Compare To Zero  relop=<=  OutDataTypeStr=boolean
  Compare To Zero3 : simulink/Logic and Bit Operations/Compare To Zero  relop=<=  OutDataTypeStr=boolean
  Constant : Constant  Value=[1 1 1 1 1]
  Constant5 : Constant
  Data Type Conversion{,1..5} (6 alike) : DataTypeConversion
  Demux{,1..5} (6 alike) : Demux  Outputs=5
  Efficiencies : Lookup  InputValues=[1:length(transmission.ratios)]  Table=transmission.trq_eff  LookUpMeth=Use Input Nearest
  Full load curve : Lookup  InputValues=em.speed  Table=em.trq  LookUpMeth=Interpolation-Use End Values
  Gear change recommendation : Subsystem
  Gearing : Lookup  InputValues=[1:length(transmission.ratios)]  Table=transmission.ratios  LookUpMeth=Use Input Nearest
  M*=M/i eta : Product  Inputs=/*/
  Mux : Mux  Inputs=5
  Saturation{,1..3} (4 alike) : Saturate  UpperLimit=length(transmission.ratios)  LowerLimit=0
  Sum1 : Sum  Inputs=-+|
  Sum2 : Sum  Inputs=-+|
  Sum3 : Sum  Inputs=+-|
  Switch : Switch  Criteria=u2 > Threshold  Threshold=0.06
  Terminator1 : Terminator
  Terminator2 : Terminator
  Terminator3 : Terminator
  engine speed max : Constant  Value=em.n_max
  n*=n*i : Product  Inputs=**
  standstill : Constant  Value=0
  torque resever : Gain  Gain=0.8
  reccommend_down_2higher : Outport  VectorParamsAs1DForOutWhenUnconnected=off
  reccommend_down_1higher : Outport  Port=2  VectorParamsAs1DForOutWhenUnconnected=off
  reccommend_down_now : Outport  Port=3  VectorParamsAs1DForOutWhenUnconnected=off
  reccommend_down_1lower : Outport  Port=4  VectorParamsAs1DForOutWhenUnconnected=off
  reccommend_down_2lower : Outport  Port=5  VectorParamsAs1DForOutWhenUnconnected=off
  reccommend_up_2higher : Outport  Port=6  VectorParamsAs1DForOutWhenUnconnected=off
  reccommend_up_1higher : Outport  Port=7  VectorParamsAs1DForOutWhenUnconnected=off
  reccommend_up_now : Outport  Port=8  VectorParamsAs1DForOutWhenUnconnected=off
  reccommend_up_1lower : Outport  Port=9  VectorParamsAs1DForOutWhenUnconnected=off
  reccommend_up_2lower : Outport  Port=10  VectorParamsAs1DForOutWhenUnconnected=off
  check_n_min_2higher : Outport  Port=11  VectorParamsAs1DForOutWhenUnconnected=off
  check_n_min_1higher : Outport  Port=12  VectorParamsAs1DForOutWhenUnconnected=off
  check_n_min_now : Outport  Port=13  VectorParamsAs1DForOutWhenUnconnected=off
  check_n_min_1lower : Outport  Port=14  VectorParamsAs1DForOutWhenUnconnected=off
  check_n_min_2lower : Outport  Port=15  VectorParamsAs1DForOutWhenUnconnected=off
  check_n_max_2higher : Outport  Port=16  VectorParamsAs1DForOutWhenUnconnected=off
  check_n_max_1higher : Outport  Port=17  VectorParamsAs1DForOutWhenUnconnected=off
  check_n_max_now : Outport  Port=18  VectorParamsAs1DForOutWhenUnconnected=off
  check_n_max_1lower : Outport  Port=19  VectorParamsAs1DForOutWhenUnconnected=off
  check_n_max_2lower : Outport  Port=20  VectorParamsAs1DForOutWhenUnconnected=off
  check_M_max_2higher : Outport  Port=21  VectorParamsAs1DForOutWhenUnconnected=off
  check_M_max_1higher : Outport  Port=22  VectorParamsAs1DForOutWhenUnconnected=off
  check_M_max_now : Outport  Port=23  VectorParamsAs1DForOutWhenUnconnected=off
  check_M_max_1lower : Outport  Port=24  VectorParamsAs1DForOutWhenUnconnected=off
  check_M_max_2lower : Outport  Port=25  VectorParamsAs1DForOutWhenUnconnected=off
  check_torque_reseve_2higher : Outport  Port=26  VectorParamsAs1DForOutWhenUnconnected=off
  check_torque_reseve_2lower : Outport  Port=27  VectorParamsAs1DForOutWhenUnconnected=off
  wires:
  Gear/1 -> 1 gear higher/1, Mux/3, 1 gear lower/1, 2 gears lower/1, 2 gears higher/1  "Current gear"
  n*=n*i/1 -> Full load curve/1, Sum1/2, Sum3/2, Gear change recommendation/2(n_ICE [rpm])  "n_gearbox_in [1/min]"
  n_Getr_out [1/min]/1 -> n*=n*i/2
  Efficiencies/1 -> M*=M/i eta/1
  M_Getr_out [Nm]/1 -> M*=M/i eta/2
  2 gears higher/1 -> Saturation/1
  1 gear higher/1 -> Saturation1/1
  Mux/1 -> Efficiencies/1, Gearing/1
  Demux/1 -> reccommend_down_2higher/1
  Demux/2 -> reccommend_down_1higher/1
  Demux/3 -> reccommend_down_now/1
  Demux2/1 -> check_torque_reseve_2higher/1
  Demux2/2 -> Terminator2/1
  Demux2/3 -> Terminator1/1
  Demux1/1 -> check_n_min_2higher/1
  Demux1/2 -> check_n_min_1higher/1
  Demux1/3 -> check_n_min_now/1
  Gearing/1 -> n*=n*i/1, M*=M/i eta/3
  Saturation/1 -> Mux/1
  Saturation1/1 -> Mux/2
  1 gear lower/1 -> Saturation2/1
  Saturation2/1 -> Mux/4
  2 gears lower/1 -> Saturation3/1
  Saturation3/1 -> Mux/5
  Demux2/4 -> Terminator3/1
  Demux2/5 -> check_torque_reseve_2lower/1
  Demux/5 -> reccommend_down_2lower/1
  Demux/4 -> reccommend_down_1lower/1
  Demux1/4 -> check_n_min_1lower/1
  Demux1/5 -> check_n_min_2lower/1
  Demux4/1 -> reccommend_up_2higher/1
  Demux4/2 -> reccommend_up_1higher/1
  Demux4/3 -> reccommend_up_now/1
  Demux4/5 -> reccommend_up_2lower/1
  Demux4/4 -> reccommend_up_1lower/1
  Gear change recommendation/1(recommend_down) -> Data Type Conversion1/1
  Full load curve/1 -> torque resever/1
  torque resever/1 -> Sum2/1
  Sum2/1 -> Compare To Zero2/1
  Compare To Zero2/1 -> Data Type Conversion5/1
  Sum3/1 -> Compare To Zero3/1
  standstill/1 -> Sum3/1
  Compare To Zero3/1 -> Data Type Conversion3/1
  Gear change recommendation/2(recommend_up) -> Data Type Conversion2/1
  Demux3/1 -> check_n_max_2higher/1
  Demux3/2 -> check_n_max_1higher/1
  Demux3/3 -> check_n_max_now/1
  Demux3/4 -> check_n_max_1lower/1
  Demux3/5 -> check_n_max_2lower/1
  Sum1/1 -> Compare To Zero1/1
  engine speed max/1 -> Sum1/1
  Demux5/1 -> check_M_max_2higher/1
  Demux5/2 -> check_M_max_1higher/1
  Demux5/3 -> check_M_max_now/1
  Demux5/4 -> check_M_max_1lower/1
  Demux5/5 -> check_M_max_2lower/1
  Data Type Conversion1/1 -> Demux/1
  Data Type Conversion2/1 -> Demux4/1
  Data Type Conversion3/1 -> Demux1/1
  Data Type Conversion4/1 -> Demux3/1
  Data Type Conversion/1 -> Demux5/1
  Data Type Conversion5/1 -> Demux2/1
  Constant/1 -> Data Type Conversion/1
  M*=M/i eta/1 -> Gear change recommendation/1(M_ICE [Nm]), Sum2/2  "M_gearbox_in [Nm]M"
  delta_v/1 -> Gear change recommendation/3(delta_v)
  v_target [m/s]/1 -> Gear change recommendation/4(v_target [m/s])
  Constant5/1 -> Switch/1
  Switch/1 -> Data Type Conversion4/1
  Compare To Zero1/1 -> Switch/3
  alpha/1 -> Switch/2, Gear change recommendation/5(alpha [rad])

== system HDVSim_BEV_Truck/Transmission/Torque flow through the transmission ==
  note: Outgoing torque from the transmission
  note: Rotational speed before and after the transmission
  M_gearbox_in [Nm] : Inport
  n_gearbox_out [1/min] : Inport  Port=2
  Gear : Inport  Port=3
  Divide : Product  Inputs=/
  Efficiencies : Lookup  InputValues=[1:length(transmission.ratios)]  Table=transmission.trq_eff  LookUpMeth=Use Input Nearest
  Gearing : Lookup  InputValues=[1:length(transmission.ratios)]  Table=transmission.ratios  LookUpMeth=Use Input Nearest
  M_Mot >= 0? : Switch  ZeroCross=off
  Product : Product  Inputs=***  RndMeth=Zero
  Rotating mass : Lookup  InputValues=[1:length(transmission.ratios)]  Table=transmission.lamda  LookUpMeth=Use Input Nearest
  Subsystem : Subsystem  Commented=on
  n*=n*i : Product  Inputs=**
  n_gearbox_in [1/min] : Outport  VectorParamsAs1DForOutWhenUnconnected=off
  M_gearbox_out [Nm] : Outport  Port=2  VectorParamsAs1DForOutWhenUnconnected=off
  i_gearbox : Outport  Port=3  VectorParamsAs1DForOutWhenUnconnected=off
  tag scope: Eta_Transmission=global, lamda=global
  wires:
  Divide/1 -> M_Mot >= 0?/3
  Rotating mass/1 -> [lamda]  "lambda"
  Efficiencies/1 -> Divide/1, M_Mot >= 0?/1  "Eta_Gear"
  Gear/1 -> Rotating mass/1, Gearing/1, Efficiencies/1
  Product/1 -> M_gearbox_out [Nm]/1
  n*=n*i/1 -> n_gearbox_in [1/min]/1
  Gearing/1 -> n*=n*i/1, i_gearbox/1, Product/3  "i_Gear"
  M_gearbox_in [Nm]/1 -> M_Mot >= 0?/2, Product/2
  n_gearbox_out [1/min]/1 -> n*=n*i/2
  M_Mot >= 0?/1 -> [Eta_Transmission], Product/1

== system HDVSim_BEV_Truck/Transmission/ZKU ==
  Gear : Inport
  Compare : simulink/Logic and Bit Operations/Compare To Zero  relop=>=  OutDataTypeStr=uint8  ZeroCross=off
  Constant : Constant  Value=-1
  Constant1 : Constant  Value=0
  Data Type Conversion : DataTypeConversion
  Derivative : Derivative
  Integrator : Integrator  ExternalReset=either  InitialCondition=transmission.shift_time
  Manual Switch : ManualSwitch
  tag scope: ZKU=global
  wires:
  Constant/1 -> Integrator/1
  Derivative/1 -> Integrator/2
  Integrator/1 -> Compare/1
  Compare/1 -> Data Type Conversion/1
  Data Type Conversion/1 -> [ZKU]
  Constant1/1 -> Manual Switch/2
  Gear/1 -> Manual Switch/1
  Manual Switch/1 -> Derivative/1

== system HDVSim_BEV_Truck/Vehicle/Driving resistances without acceleration ==
  alpha [rad] : Inport
  v [m/s] : Inport  Port=2
  Add : Sum  Inputs=+++
  Drag : Subsystem
  Gradient resistance : Subsystem
  Rolling resistance : Subsystem
  F_W [N] : Outport  VectorParamsAs1DForOutWhenUnconnected=off
  tag scope: Air_drag=global, Rolling_drag=global
  wires:
  Drag/1(F_drag [N]) -> [Air_drag], Add/2
  Rolling resistance/1(F_Roll [N]) -> Add/1, [Rolling_drag]
  Add/1 -> F_W [N]/1
  v [m/s]/1 -> Drag/1(v [m/s])
  Gradient resistance/1(F_slope [N]) -> Add/3
  alpha [rad]/1 -> Gradient resistance/1(alpha [rad]), Rolling resistance/1(alpha [rad])

== system HDVSim_BEV_Truck/Active cruise control1/Estimate acceleration/Driving resistance without acceleration ==
  v [m/s] : Inport
  alpha [rad] : Inport  Port=2
  Add : Sum  Inputs=+++
  "Drag " : Subsystem
  Gradient resistance : Subsystem
  Rolling resistance : Subsystem
  F_x (resist) [N] : Outport  VectorParamsAs1DForOutWhenUnconnected=off
  wires:
  "Drag "/1(F_drag [N]) -> Add/2
  Rolling resistance/1(F_Roll [N]) -> Add/1
  Add/1 -> F_x (resist) [N]/1  "F_W"
  v [m/s]/1 -> "Drag "/1(v [m/s])
  Gradient resistance/1(F_slope [N]) -> Add/3
  alpha [rad]/1 -> Gradient resistance/1(alpha [rad]), Rolling resistance/1(alpha [rad])

== system HDVSim_BEV_Truck/Active cruise control2/Estimate acceleration/Driving resistance without acceleration ==
  v [m/s] : Inport
  alpha [rad] : Inport  Port=2
  Add : Sum  Inputs=+++
  "Drag " : Subsystem
  Gradient resistance : Subsystem
  Rolling resistance : Subsystem
  F_x (resist) [N] : Outport  VectorParamsAs1DForOutWhenUnconnected=off
  wires:
  "Drag "/1(F_drag [N]) -> Add/2
  Rolling resistance/1(F_Roll [N]) -> Add/1
  Add/1 -> F_x (resist) [N]/1  "F_W"
  v [m/s]/1 -> "Drag "/1(v [m/s])
  Gradient resistance/1(F_slope [N]) -> Add/3
  alpha [rad]/1 -> Gradient resistance/1(alpha [rad]), Rolling resistance/1(alpha [rad])

== system HDVSim_BEV_Truck/Active cruise control_old/Estimate acceleration/Fahrwiderstaende ohne Beschleunigung ==
  v [m/s] : Inport
  alpha [rad] : Inport  Port=2
  Add : Sum  Inputs=+++
  drag - Luftwiderstand : Subsystem
  grade resistance - Steigungswiderstand : Subsystem
  rolling resistance - Rollwiderstand : Subsystem
  F_x (Widerstand) [N] : Outport  VectorParamsAs1DForOutWhenUnconnected=off
  wires:
  drag - Luftwiderstand/1(F_Luft [N]) -> Add/2
  rolling resistance - Rollwiderstand/1(F_Roll [N]) -> Add/1
  Add/1 -> F_x (Widerstand) [N]/1  "F_W"
  v [m/s]/1 -> drag - Luftwiderstand/1(v [m/s])
  grade resistance - Steigungswiderstand/1(F_Steig [N]) -> Add/3
  alpha [rad]/1 -> grade resistance - Steigungswiderstand/1(alpha [rad]), rolling resistance - Rollwiderstand/1(alpha [rad])

== system HDVSim_BEV_Truck/Transmission/Determine when shifting occurs/Gear change recommendation ==
  note: Gear change commands
  M_ICE [Nm] : Inport
  n_ICE [rpm] : Inport  Port=2
  delta_v : Inport  Port=3
  v_target [m/s] : Inport  Port=4
  alpha [rad] : Inport  Port=5
  Constant1 : Constant  Value=0
  Constant3 : Constant  Value=em.shift_parameter.n2
  Constant5 : Constant  Value=em.shift_parameter.n6
  M_max [Nm] : Constant  Value=em.M_max
  Switch : Switch  Criteria=u2 > Threshold  Threshold=0.06
  recommend_down_calcbsfc1 : Subsystem
  recommend_up_calc_bsfc1 : Subsystem
  recommend_down : Outport  VectorParamsAs1DForOutWhenUnconnected=off
  recommend_up : Outport  Port=2  VectorParamsAs1DForOutWhenUnconnected=off
  wires:
  M_max [Nm]/1 -> recommend_up_calc_bsfc1/5(M_max [Nm])  "M_max"
  n_ICE [rpm]/1 -> recommend_up_calc_bsfc1/4(n), recommend_down_calcbsfc1/1(n_ICE [rpm])
  M_ICE [Nm]/1 -> recommend_up_calc_bsfc1/1(M)
  recommend_down_calcbsfc1/1(Out1) -> recommend_down/1
  Constant3/1 -> recommend_up_calc_bsfc1/3(n_2), recommend_down_calcbsfc1/2(shift_parameter.n_2)
  Constant5/1 -> recommend_up_calc_bsfc1/2(n_6)
  delta_v/1 -> recommend_down_calcbsfc1/3(delta_v)
  v_target [m/s]/1 -> recommend_up_calc_bsfc1/6(v_target [m/s])
  Constant1/1 -> Switch/1
  recommend_up_calc_bsfc1/1(recommend_up) -> Switch/3
  Switch/1 -> recommend_up/1
  alpha [rad]/1 -> Switch/2

== system HDVSim_BEV_Truck/Transmission/Torque flow through the transmission/Subsystem ==
  M_in : Inport
  z : Inport  Port=2
  n_in : Inport  Port=3
  M_out : Outport  VectorParamsAs1DForOutWhenUnconnected=off
  i : Outport  Port=2  VectorParamsAs1DForOutWhenUnconnected=off
  n_out : Outport  Port=3  VectorParamsAs1DForOutWhenUnconnected=off
  lambda : Outport  Port=4  VectorParamsAs1DForOutWhenUnconnected=off

== system HDVSim_BEV_Truck/Vehicle/Driving resistances without acceleration/Drag ==
  note: F_Drag = 0.5 * V^2 * rho * A * c_d
  v [m/s] : Inport
  A : Constant  Value=vehicle.frontal_area
  Product2 : Product  Inputs=4  RndMeth=Zero
  c_d : Constant  Value=vehicle.air_drag_coeff
  gain2 : Gain  Gain=0.5
  rho : Constant  Value=ambient.air_density
  v² : Math  Operator=square  SaturateOnIntegerOverflow=on
  F_drag [N] : Outport  VectorParamsAs1DForOutWhenUnconnected=off
  wires:
  v²/1 -> Product2/1
  gain2/1 -> F_drag [N]/1
  v [m/s]/1 -> v²/1
  rho/1 -> Product2/2
  A/1 -> Product2/3
  c_d/1 -> Product2/4
  Product2/1 -> gain2/1

== system HDVSim_BEV_Truck/Vehicle/Driving resistances without acceleration/Gradient resistance ==
  note: F_slope = (m_tot * g) * sin(alpha)
  alpha [rad] : Inport
  Add : Sum
  Cargo weight : Constant  Value=vehicle.payload
  Product7 : Product  RndMeth=Zero
  Trigonometric Function : Trigonometry
  Vehicle weight : Constant  Value=vehicle.mass
  g : Gain  Gain=ambient.gravity
  F_slope [N] : Outport  VectorParamsAs1DForOutWhenUnconnected=off
  wires:
  alpha [rad]/1 -> Trigonometric Function/1
  Trigonometric Function/1 -> Product7/2
  Product7/1 -> F_slope [N]/1
  g/1 -> Product7/1
  Vehicle weight/1 -> Add/1
  Cargo weight/1 -> Add/2
  Add/1 -> g/1

== system HDVSim_BEV_Truck/Vehicle/Driving resistances without acceleration/Rolling resistance ==
  note: F_Roll = (m_tot * g) * mu * cos(alpha)
  alpha [rad] : Inport
  Add1 : Sum
  Cargo weight : Constant  Value=vehicle.payload
  Product7 : Product  Inputs=3  RndMeth=Zero
  Rolling friction coefficient : Constant  Value=tires.roll_drag_coeff.total
  Trigonometric Function : Trigonometry  Operator=cos
  Vehicle weight : Constant  Value=vehicle.mass
  g : Gain  Gain=ambient.gravity
  F_Roll [N] : Outport  VectorParamsAs1DForOutWhenUnconnected=off
  wires:
  alpha [rad]/1 -> Trigonometric Function/1
  Product7/1 -> F_Roll [N]/1
  Rolling friction coefficient/1 -> Product7/3
  Trigonometric Function/1 -> Product7/1
  g/1 -> Product7/2
  Vehicle weight/1 -> Add1/1
  Cargo weight/1 -> Add1/2
  Add1/1 -> g/1

== system HDVSim_BEV_Truck/Active cruise control1/Estimate acceleration/Driving resistance without acceleration/Drag  ==
  note: F_Drag = 0.5 * V^2 * rho * A * c_d
  v [m/s] : Inport
  A : Constant  Value=vehicle.frontal_area
  Product2 : Product  Inputs=4  RndMeth=Zero
  c_d : Constant  Value=vehicle.air_drag_coeff(end)
  gain2 : Gain  Gain=0.5
  rho : Constant  Value=ambient.air_density
  v² : Math  Operator=square  SaturateOnIntegerOverflow=on
  F_drag [N] : Outport  VectorParamsAs1DForOutWhenUnconnected=off
  wires:
  v²/1 -> Product2/1
  gain2/1 -> F_drag [N]/1
  v [m/s]/1 -> v²/1
  rho/1 -> Product2/2
  A/1 -> Product2/3
  Product2/1 -> gain2/1
  c_d/1 -> Product2/4

== system HDVSim_BEV_Truck/Active cruise control1/Estimate acceleration/Driving resistance without acceleration/Gradient resistance ==
  note: F_slope = (m_tot * g) * sin(alpha)
  alpha [rad] : Inport
  Add : Sum
  Constant1 : Constant  Value=vehicle.payload
  Constant2 : Constant  Value=vehicle.mass
  Product7 : Product  RndMeth=Zero
  Trigonometric Function : Trigonometry
  g : Gain  Gain=ambient.gravity
  F_slope [N] : Outport  VectorParamsAs1DForOutWhenUnconnected=off
  wires:
  alpha [rad]/1 -> Trigonometric Function/1
  Trigonometric Function/1 -> Product7/2
  Product7/1 -> F_slope [N]/1
  g/1 -> Product7/1
  Constant2/1 -> Add/1
  Constant1/1 -> Add/2
  Add/1 -> g/1

== system HDVSim_BEV_Truck/Active cruise control1/Estimate acceleration/Driving resistance without acceleration/Rolling resistance ==
  note: F_Roll = (m_tot * g) * mu * cos(alpha)
  alpha [rad] : Inport
  Add1 : Sum
  Constant1 : Constant  Value=vehicle.payload
  Constant5 : Constant  Value=tires.roll_drag_coeff.total
  Constant8 : Constant  Value=vehicle.mass
  Product7 : Product  Inputs=3  RndMeth=Zero
  Trigonometric Function : Trigonometry  Operator=cos
  g : Gain  Gain=ambient.gravity
  F_Roll [N] : Outport  VectorParamsAs1DForOutWhenUnconnected=off
  wires:
  alpha [rad]/1 -> Trigonometric Function/1
  Product7/1 -> F_Roll [N]/1
  Constant5/1 -> Product7/3
  Trigonometric Function/1 -> Product7/1
  g/1 -> Product7/2
  Constant8/1 -> Add1/1
  Constant1/1 -> Add1/2
  Add1/1 -> g/1

== system HDVSim_BEV_Truck/Active cruise control2/Estimate acceleration/Driving resistance without acceleration/Drag  ==
  note: F_Drag = 0.5 * V^2 * rho * A * c_d
  v [m/s] : Inport
  A : Constant  Value=vehicle.frontal_area
  Product2 : Product  Inputs=4  RndMeth=Zero
  c_d : Constant  Value=vehicle.air_drag_coeff(end)
  gain2 : Gain  Gain=0.5
  rho : Constant  Value=ambient.air_density
  v² : Math  Operator=square  SaturateOnIntegerOverflow=on
  F_drag [N] : Outport  VectorParamsAs1DForOutWhenUnconnected=off
  wires:
  v²/1 -> Product2/1
  gain2/1 -> F_drag [N]/1
  v [m/s]/1 -> v²/1
  rho/1 -> Product2/2
  A/1 -> Product2/3
  Product2/1 -> gain2/1
  c_d/1 -> Product2/4

== system HDVSim_BEV_Truck/Active cruise control2/Estimate acceleration/Driving resistance without acceleration/Gradient resistance ==
  note: F_slope = (m_tot * g) * sin(alpha)
  alpha [rad] : Inport
  Add : Sum
  Constant1 : Constant  Value=vehicle.payload
  Constant2 : Constant  Value=vehicle.mass
  Product7 : Product  RndMeth=Zero
  Trigonometric Function : Trigonometry
  g : Gain  Gain=ambient.gravity
  F_slope [N] : Outport  VectorParamsAs1DForOutWhenUnconnected=off
  wires:
  alpha [rad]/1 -> Trigonometric Function/1
  Trigonometric Function/1 -> Product7/2
  Product7/1 -> F_slope [N]/1
  g/1 -> Product7/1
  Constant2/1 -> Add/1
  Constant1/1 -> Add/2
  Add/1 -> g/1

== system HDVSim_BEV_Truck/Active cruise control2/Estimate acceleration/Driving resistance without acceleration/Rolling resistance ==
  note: F_Roll = (m_tot * g) * mu * cos(alpha)
  alpha [rad] : Inport
  Add1 : Sum
  Constant1 : Constant  Value=vehicle.payload
  Constant5 : Constant  Value=tires.roll_drag_coeff.total
  Constant8 : Constant  Value=vehicle.mass
  Product7 : Product  Inputs=3  RndMeth=Zero
  Trigonometric Function : Trigonometry  Operator=cos
  g : Gain  Gain=ambient.gravity
  F_Roll [N] : Outport  VectorParamsAs1DForOutWhenUnconnected=off
  wires:
  alpha [rad]/1 -> Trigonometric Function/1
  Product7/1 -> F_Roll [N]/1
  Constant5/1 -> Product7/3
  Trigonometric Function/1 -> Product7/1
  g/1 -> Product7/2
  Constant8/1 -> Add1/1
  Constant1/1 -> Add1/2
  Add1/1 -> g/1
